simulink model "datafusion_realdata"  (R2020b)
settings: Solver=VariableStepAuto  StartTime=0.0  StopTime=20.0  RelTol=1e-3
model workspace (MAT data in the model file):
  sample_time = 0.01
libraries: simulink x4
settings Model: Creator=tfpeng  LastModifiedBy=tfpeng

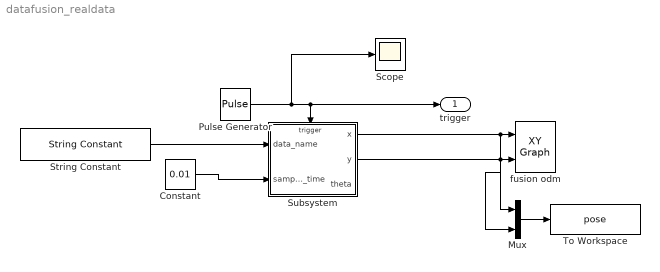
== system datafusion_realdata ==
  Constant : Constant  Value=0.01
  Mux : Mux  Inputs=2
  Pulse Generator : DiscretePulseGenerator  PulseType=Time based  Period=0.001  PulseWidth=50
  Scope : Scope
  String Constant : StringConstant  String="\"debug_output_2023-09-19_08:02:57.dat\""
  Subsystem : Subsystem
  To Workspace : ToWorkspace  VariableName=pose  SampleTime=-1
      settings: Save2DSignal=2-D array (concatenate along first dimension)
  fusion odm : simulink/Sinks/XY Graph  xmin=-5  xmax=5  ymin=-5  ymax=5  st=-1
  trigger : Outport
  wires:
  Pulse Generator/1 -> Scope/1, trigger/1, Subsystem/Trigger
  String Constant/1 -> Subsystem/1(data_name)
  Constant/1 -> Subsystem/2(sample_time)
  Subsystem/2(y) -> Mux/2, fusion odm/2
  Subsystem/1(x) -> Mux/1, fusion odm/1
  Mux/1 -> To Workspace/1

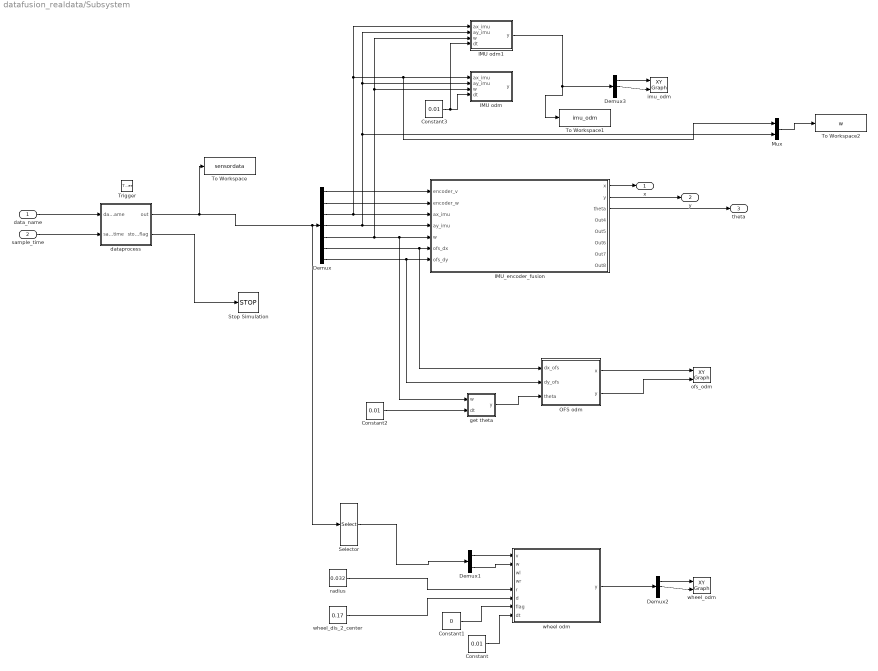
== system datafusion_realdata/Subsystem ==
  data_name : Inport
  sample_time : Inport  Port=2
  Trigger : TriggerPort  VariantControl=Variant  PortDimensions=1
  Constant : Constant  Value=0.01
  Constant1 : Constant  Value=0
  Constant2 : Constant  Value=0.01
  Constant3 : Constant  Value=0.01
  Demux : Demux  Outputs=7
  Demux1 : Demux  Outputs=2
  Demux2 : Demux  Outputs=3
  Demux3 : Demux  Outputs=3
  IMU odm : MATLAB Function  TreatAsAtomicUnit=on
  IMU odm1 : MATLAB Function  TreatAsAtomicUnit=on
  IMU_encoder_fusion : Subsystem
  Mux : Mux  Inputs=2
  OFS odm : Subsystem
  Selector : Selector  InputPortWidth=7  IndexOptions=Index vector (dialog)  Indices=[1 2]  OutputSizes=1
  Stop Simulation : Stop
  To Workspace : ToWorkspace  VariableName=sensordata  SampleTime=-1
      settings: Save2DSignal=2-D array (concatenate along first dimension)
  To Workspace1 : ToWorkspace  VariableName=imu_odm  SampleTime=-1
      settings: Save2DSignal=2-D array (concatenate along first dimension)
  To Workspace2 : ToWorkspace  VariableName=w  SampleTime=-1
      settings: Save2DSignal=2-D array (concatenate along first dimension)
  dataprocess : MATLAB Function  TreatAsAtomicUnit=on
  get theta : MATLAB Function  TreatAsAtomicUnit=on
  imu_odm : simulink/Sinks/XY Graph  xmin=-10  xmax=10  ymin=-10  ymax=10  st=-1
  ofs_odm : simulink/Sinks/XY Graph  xmin=-5  xmax=5  ymin=-5  ymax=5  st=-1
  radius : Constant  Value=0.032
  wheel odm : MATLAB Function  TreatAsAtomicUnit=on
  wheel_dis_2_center : Constant  Value=0.17
  wheel_odm : simulink/Sinks/XY Graph  xmin=-5  xmax=5  ymin=-5  ymax=5  st=-1
  x : Outport
  y : Outport  Port=2
  theta : Outport  Port=3
  wires:
  data_name/1 -> dataprocess/1(data_name)
  sample_time/1 -> dataprocess/2(sample_time)
  Demux/2 -> IMU_encoder_fusion/2(encoder_w)
  Demux/4 -> IMU odm1/2(ay_imu), IMU odm/2(ay_imu), Mux/2, IMU_encoder_fusion/4(ay_imu)
  Demux/3 -> IMU odm1/1(ax_imu), Mux/1, IMU odm/1(ax_imu), IMU_encoder_fusion/3(ax_imu)
  Demux/7 -> OFS odm/2(dy_ofs), IMU_encoder_fusion/7(ofs_dy)
  dataprocess/1(out) -> To Workspace/1, Selector/1, Demux/1
  Demux/6 -> OFS odm/1(dx_ofs), IMU_encoder_fusion/6(ofs_dx)
  Demux/1 -> IMU_encoder_fusion/1(encoder_v)
  IMU_encoder_fusion/1(x) -> x/1
  IMU_encoder_fusion/2(y) -> y/1
  IMU_encoder_fusion/3(theta) -> theta/1
  dataprocess/2(stop_flag) -> Stop Simulation/1
  wheel_dis_2_center/1 -> wheel odm/6(d)
  radius/1 -> wheel odm/5(r)
  Selector/1 -> Demux1/1
  Demux1/1 -> wheel odm/1(v)
  Demux1/2 -> wheel odm/2(w)
  Constant/1 -> wheel odm/8(dt)
  wheel odm/1(y) -> Demux2/1
  Demux2/1 -> wheel_odm/1
  Demux2/2 -> wheel_odm/2
  Constant1/1 -> wheel odm/7(flag)
  Constant2/1 -> get theta/2(dt)
  OFS odm/1(x) -> ofs_odm/1
  OFS odm/2(y) -> ofs_odm/2
  Demux/5 -> IMU odm1/3(w), IMU odm/3(w), get theta/1(w), IMU_encoder_fusion/5(w)
  get theta/1(y) -> OFS odm/3(theta)
  Constant3/1 -> IMU odm1/4(dt), IMU odm/4(dt)
  Demux3/2 -> imu_odm/2
  Demux3/1 -> imu_odm/1
  Mux/1 -> To Workspace2/1
  IMU odm1/1(y) -> To Workspace1/1, Demux3/1

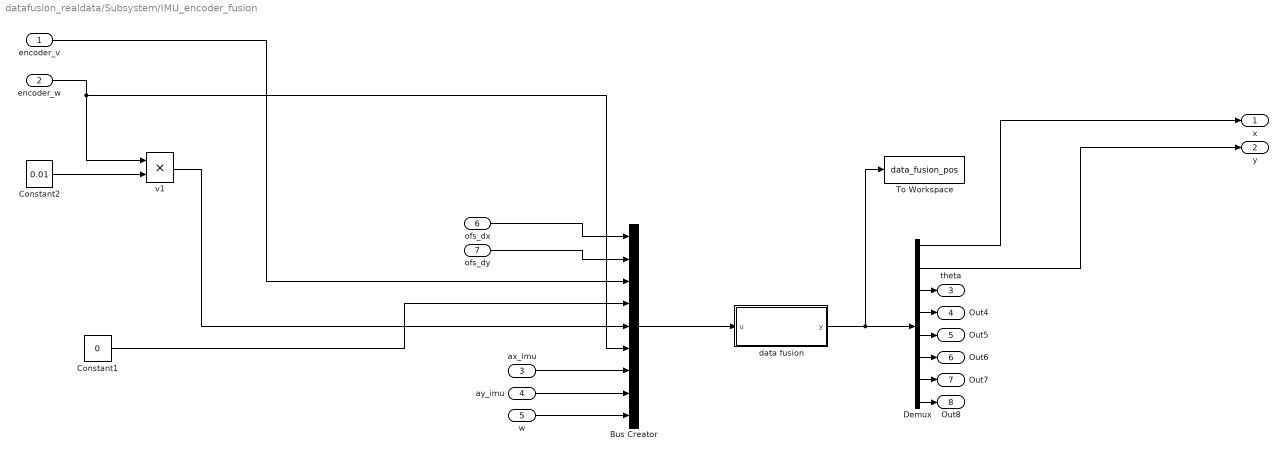
== system datafusion_realdata/Subsystem/IMU_encoder_fusion ==
  encoder_v : Inport
  encoder_w : Inport  Port=2
  ax_imu : Inport  Port=3
  ay_imu : Inport  Port=4
  w : Inport  Port=5
  ofs_dx : Inport  Port=6
  ofs_dy : Inport  Port=7
  Bus Creator : BusCreator  Inputs=9
  Constant1 : Constant  Value=0
  Constant2 : Constant  Value=0.01
  Demux : Demux  Outputs=8
  To Workspace : ToWorkspace  VariableName=data_fusion_pos  SampleTime=-1
      settings: Save2DSignal=2-D array (concatenate along first dimension)
  data fusion : Subsystem  TreatAsAtomicUnit=on
  v1 : Product
  x : Outport
  y : Outport  Port=2
  theta : Outport  Port=3
  Out4 : Outport  Port=4
  Out5 : Outport  Port=5
  Out6 : Outport  Port=6
  Out7 : Outport  Port=7
  Out8 : Outport  Port=8
  wires:
  Demux/7 -> Out7/1
  Demux/8 -> Out8/1
  Demux/2 -> y/1
  ax_imu/1 -> Bus Creator/7
  Demux/3 -> theta/1
  w/1 -> Bus Creator/9
  encoder_v/1 -> Bus Creator/3
  ay_imu/1 -> Bus Creator/8
  data fusion/1(y) -> To Workspace/1, Demux/1
  Demux/4 -> Out4/1
  Demux/1 -> x/1
  Demux/5 -> Out5/1
  Bus Creator/1 -> data fusion/1(u)
  Demux/6 -> Out6/1
  ofs_dx/1 -> Bus Creator/1
  ofs_dy/1 -> Bus Creator/2
  Constant2/1 -> v1/2
  encoder_w/1 -> Bus Creator/6, v1/1
  v1/1 -> Bus Creator/5
  Constant1/1 -> Bus Creator/4

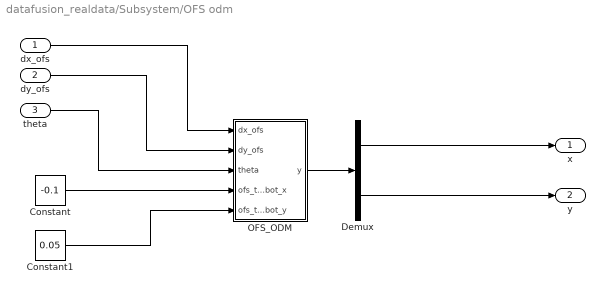
== system datafusion_realdata/Subsystem/OFS odm ==
  dx_ofs : Inport
  dy_ofs : Inport  Port=2
  theta : Inport  Port=3
  Constant : Constant  Value=-0.1
  Constant1 : Constant  Value=0.05
  Demux : Demux  Outputs=2
  OFS_ODM : MATLAB Function  TreatAsAtomicUnit=on
  x : Outport
  y : Outport  Port=2
  wires:
  Demux/2 -> y/1
  Demux/1 -> x/1
  theta/1 -> OFS_ODM/3(theta)
  dx_ofs/1 -> OFS_ODM/1(dx_ofs)
  OFS_ODM/1(y) -> Demux/1
  dy_ofs/1 -> OFS_ODM/2(dy_ofs)
  Constant/1 -> OFS_ODM/4(ofs_to_robot_x)
  Constant1/1 -> OFS_ODM/5(ofs_to_robot_y)

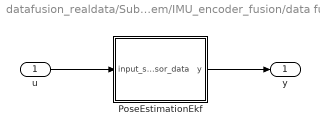
== system datafusion_realdata/Subsystem/IMU_encoder_fusion/data fusion ==
  u : Inport
  PoseEstimationEkf : MATLAB Function  TreatAsAtomicUnit=on
  y : Outport
  wires:
  u/1 -> PoseEstimationEkf/1(input_sensor_data)
  PoseEstimationEkf/1(y) -> y/1

== matlab function datafusion_realdata/Subsystem/wheel odm ==
  data: v input; y output; w input; wl input; wr input; r input; d input; flag input; dt input
function y = wheelodm( v,w,wl,wr,r,d,flag,dt)
persistent pos last_pos;
if isempty(pos)
   pos=zeros(3,1);%x,y,theta 
   last_pos=pos;
end
if flag==0
   %use v,w 
   vx=v*cos(pos(3));
   vy=v*sin(pos(3));
   dx=vx*dt;
   dy=vy*dt;
   dtheta=w*dt;
   pos=pos+[dx;dy;dtheta];
    
else
    %use wl,wr
    pos=zeros(3,1);%x,y,theta
    
end
y = pos;

== matlab function datafusion_realdata/Subsystem/dataprocess ==
  data: data_name input; out output; sample_time input; stop_flag output
function [out,stop_flag]= realdata_read(data_name,sample_time)
coder.extrinsic('realdata_read_callback');
out=[0,0,0,0,0,0,0];
stop_flag=0;
out=realdata_read_callback(data_name,sample_time);
if sum(out)==-7
    stop_flag=1;
end
% persistent fid;
% filepath="/home/tfpeng/work/other/TFwork/code/mat/car_simulation/";
% if isempty(fid)
%     fid=fopen(filepath+data_name,'r');
% end
% starttim=0;
% wheel_data=[];
% imu_data=[];
% ofs_data=[];
% 
% while 1
%     line=fgetl(fid);
%     newarr=split(line,': ');
%     rawdataarr=split(newarr(2)," ");
%     sensor_type=newarr{1};
%     rawdata=str2double(rawdataarr);
%     tim=rawdata(1);
%     if starttim==0
%         starttim=tim;
%     elseif contains(sensor_type,"wheel")
%        wheel_data=[wheel_data;[rawdata(1),rawdata(2)]];
%     elseif contains(sensor_type,"imu")
%        imu_data=[imu_data;[rawdata(1),rawdata(2),rawdata(3),rawdata(4),rawdata(5),rawdata(6)]]
%     elseif contains(sensor_type,"ofs")
%        ofs_data=[ofs_data;[rawdata(1),rawdata(2),rawdata(3),rawdata(4),rawdata(5)]]
%     end
%     
%     
%     if tim-starttim>=sample_time
%        break; 
%     end
%     
% end
% wheel_data_out=mean(wheel_data,1);
% imu_data_out=mean(imu_data,1);
% ofs_data_out=mean(ofs_data,1);

% out=[wheel_data_out,imu_data_out,ofs_data_out(1),ofs_data_out(2)];

== matlab function datafusion_realdata/Subsystem/IMU_encoder_fusion/data fusion/PoseEstimationEkf ==
  data: input_sensor_data input; y output
function y = PoseEstimationEkf(input_sensor_data)
persistent state_variable_current state_variable_last P Q counter vx_imu vy_imu vx_imu_last vy_imu_last;
if isempty(state_variable_current)
        state_variable_current=zeros(8,1);%[xt,yt,theta_t,vxt,vyt,wt,axt,ayt]
        state_variable_last=zeros(8,1);
        Q=diag([0.1, 0.1, 0.1,0.1, 0.1, 0.1, 0.1, 0.1]);
        P=Q;
        counter=0;
        vx_imu=0; 
        vy_imu=0;
        vx_imu_last=0;
        vy_imu_last=0;
end

%%    predict
dt=0.01;
A=[[1, 0, 0, dt, 0, 0, 0, 0]
  [0, 1, 0, 0, dt, 0, 0, 0]
  [0, 0, 1, 0, 0, dt, 0, 0]
  [0, 0, 0, 1, 0, 0, 0, 0]
  [0, 0, 0, 0, 1, 0, 0, 0]
  [0, 0, 0, 0, 0, 1, 0, 0]
  [0, 0, 0, 0, 0, 0, 0, 0]
  [0, 0, 0, 0, 0, 0, 0, 0]];
state_variable_current=A*state_variable_current;
P=A*P*A'+Q;

%%    update
theta=state_variable_current(3);
theta_last=state_variable_last(3);
vx=state_variable_current(4);
vy=state_variable_current(5);
ax=state_variable_current(7);
ay=state_variable_current(8);
dx=state_variable_current(1)-state_variable_last(1);
dy=state_variable_current(2)-state_variable_last(2);
w=state_variable_current(6);
dtheta=theta-theta_last;
v=vx*cos(theta)+vy*sin(theta);
vr=vx*sin(theta)-vy*cos(theta);
dd=sqrt(dx^2+dy^2);
% ax_imu=ax*cos(theta)+ay*sin(theta);
% ay_imu=-ax*sin(theta)+ay*cos(theta);

dx_ofs=dd*cos(dtheta/2);
dy_ofs=dd*sin(dtheta/2);

% ofs 
ofs_pos_robot=[-0.115;0.085];
rotation_matrix_last_robot_pose=[[cos(theta_last),-sin(theta_last)];
    [sin(theta_last),cos(theta_last)]];

rotation_matrix_current_robot_pose=[[cos(theta),-sin(theta)];
    [sin(theta),cos(theta)]];
last_robot_xy=[state_variable_last(1);state_variable_last(2)];
current_robot_xy=[state_variable_current(1);state_variable_current(2)];
temp2=ofs_pos_robot(1)*sin(theta)+ofs_pos_robot(2)*cos(theta);
temp3=ofs_pos_robot(1)*cos(theta)-ofs_pos_robot(2)*sin(theta);

%% all sensor data fusion ofs input distance
% H=[[cos(theta_last),sin(theta_last),cos(theta_last)*(-temp2)+temp3*sin(theta_last),0,0,0,0,0]
%    [-sin(theta_last),cos(theta_last),temp2*sin(theta_last)+temp3*cos(theta_last),0,0,0,0,0]
%    [0, 0, -vx*sin(theta)+vy*cos(theta), cos(theta), sin(theta), 0, 0, 0]
%    [0, 0, vx*cos(theta)+vy*sin(theta), sin(theta), -cos(theta), 0, 0, 0]
%    [0, 0, 1, 0, 0, 0, 0, 0]
%    [0, 0, 0, 0, 0, 1, 0, 0]
%    [0, 0, -ax*sin(theta)+ay*cos(theta), 0, 0, 0, cos(theta), sin(theta)]
%    [0, 0, -ax*cos(theta)-ay*sin(theta), 0, 0, 0, -sin(theta), cos(theta)]
%    [0, 0, 0, 0, 0, 1, 0, 0]
%    [0, 0, 1, 0, 0, 0, 0, 0]];
% Z_ofs=rotation_matrix_last_robot_pose\(current_robot_xy-last_robot_xy+rotation_matrix_current_robot_pose*ofs_pos_robot)-ofs_pos_robot;
% Z=[Z_ofs;v;vr;dtheta; w;ax_imu; ay_imu;w;dtheta];
% R = diag([0.001,0.001,0.00001,0.00001,0.00001,0.00001,0.0002,0.0002,0.0002,0.0002]);
% encoder_input_sensor_data=input_sensor_data(3:6);
% imu_input_sensor_data=[input_sensor_data(7:9);input_sensor_data(9)*dt];
% ofs_input_sensor_data=input_sensor_data(1:2);
% 
% temp_input_data=[ofs_input_sensor_data;encoder_input_sensor_data;imu_input_sensor_data];
% error=temp_input_data-Z;

%%
%% all sensor data fusion ofs input velocity
% dt=0.01;
% phi=atan(ofs_pos_robot(1)/ofs_pos_robot(2));
% l=(ofs_pos_robot'*ofs_pos_robot)^0.5;
% extern_veloctiy=[w*l*sin(phi+pi/2);w*l*sin(phi)*cos(phi+pi/2)];
% H=[[0,0,-vx*sin(theta)+vy*cos(theta)-w*l*cos(phi+pi/2-theta),cos(theta),sin(theta),l*sin(phi+pi/2-theta),0,0]
%     [0,0,-vx*cos(theta)-vy*sin(theta)+w*l*sin(phi+pi/2-theta),-sin(theta),cos(theta),l*cos(phi+pi/2-theta),0,0]
%    [0, 0, -vx*sin(theta)+vy*cos(theta), cos(theta), sin(theta), 0, 0, 0]
%    [0, 0, vx*cos(theta)+vy*sin(theta), sin(theta), -cos(theta), 0, 0, 0]
%    [0, 0, 1, 0, 0, 0, 0, 0]
%    [0, 0, 0, 0, 0, 1, 0, 0]
%    [0, 0, -ax*sin(theta)+ay*cos(theta), 0, 0, 0, cos(theta), sin(theta)]
%    [0, 0, -ax*cos(theta)-ay*sin(theta), 0, 0, 0, -sin(theta), cos(theta)]
%    [0, 0, 0, 0, 0, 1, 0, 0]
%    [0, 0, 1, 0, 0, 0, 0, 0]];
% Z_ofs=rotation_matrix_current_robot_pose\[vx;vy]+rotation_matrix_current_robot_pose*extern_veloctiy;
% Z=[Z_ofs;v;vr;dtheta; w;ax_imu; ay_imu;w;dtheta];
% R = diag([0.001,0.001,0.001,0.001,0.001,0.001,0.0002,0.0002,0.0002,0.0002]);
% encoder_input_sensor_data=input_sensor_data(3:6);
% imu_input_sensor_data=[input_sensor_data(7:9);input_sensor_data(9)*dt];
% ofs_input_sensor_data=input_sensor_data(1:2);
% 
% temp_input_data=[ofs_input_sensor_data;encoder_input_sensor_data;imu_input_sensor_data];
% error=temp_input_data-Z;
%% just wheel encoder fusion  --debug ok
% H=[[0, 0, -vx*sin(theta)+vy*cos(theta), cos(theta), sin(theta), 0, 0, 0]
%   [0, 0, vx*cos(theta)+vy*sin(theta), sin(theta), -cos(theta), 0, 0, 0]
%   [0, 0, 1, 0, 0, 0, 0, 0]
%   [0, 0, 0, 0, 0, 1, 0, 0]];
% Z=[v,vr,dtheta, w]';
% R = diag([0.001, 0.001,0.001,0.001]);
% temp_input_sensor_data=input_sensor_data(3:6);
% error=temp_input_sensor_data-Z;

%% just IMU fusion    --debug ok
% H=[[0, 0, -ax*sin(theta)+ay*cos(theta), 0, 0, 0, cos(theta), sin(theta)]
%   [0, 0, -ax*cos(theta)-ay*sin(theta), 0, 0, 0, -sin(theta), cos(theta)]
%   [0, 0, 0, 0, 0, 1, 0, 0]
%   [0, 0, 1, 0, 0, 0, 0, 0]];
% Z=[ax_imu, ay_imu,w,dtheta]';
% R = diag([0.001,0.001,0.001,0.001]);
% %[ax_imu,ay_imu,w]
% input_sensor_data=[input_sensor_data(7:9);input_sensor_data(9)*dt];
% error=input_sensor_data-Z;

%% just IMU fusion new version 
% v_imu=rotation_matrix_current_robot_pose\[vx;vy];
% temp=v_imu-[vx_imu_last;vy_imu_last];
% a_imu=temp/dt;
% ax_imu=a_imu(1,1);
% ay_imu=a_imu(2,1);
% vx_imu_last=v_imu(1,1);
% vy_imu_last=v_imu(2,1);
% H=[[0, 0, (-vx*sin(theta)+vy*cos(theta))/dt, cos(theta)/dt, sin(theta)/dt, 0, 0, 0]
%   [0, 0, -(-vx*cos(theta)-vy*sin(theta))/dt, sin(theta)/dt, -cos(theta)/dt, 0, 0, 0]
%   [0, 0, 0, 0, 0, 1, 0, 0]
%   [0, 0, 1, 0, 0, 0, 0, 0]];
% Z=[ax_imu, -ay_imu,w,dtheta]';
% R = diag([0.001,0.001,0.001,0.001]);
% %[ax_imu,ay_imu,w]
% input_sensor_data=[input_sensor_data(7:9);input_sensor_data(9)*dt];
% error=input_sensor_data-Z;

%%  IMU wheel encoder 
v_imu=rotation_matrix_current_robot_pose\[vx;vy];
temp=v_imu-[vx_imu_last;vy_imu_last];
a_imu=temp/dt;
ax_imu=a_imu(1,1);
ay_imu=a_imu(2,1);
vx_imu_last=v_imu(1,1);
vy_imu_last=v_imu(2,1);
H=[[0, 0, -vx*sin(theta)+vy*cos(theta), cos(theta), sin(theta), 0, 0, 0]
  [0, 0, vx*cos(theta)+vy*sin(theta), sin(theta), -cos(theta), 0, 0, 0]
  [0, 0, 1, 0, 0, 0, 0, 0]
  [0, 0, 0, 0, 0, 1, 0, 0]
  [0, 0, (-vx*sin(theta)+vy*cos(theta))/dt, cos(theta)/dt, sin(theta)/dt, 0, 0, 0]
  [0, 0, -(-vx*cos(theta)-vy*sin(theta))/dt, sin(theta)/dt, -cos(theta)/dt, 0, 0, 0]
  [0, 0, 0, 0, 0, 1, 0, 0]
  [0, 0, 1, 0, 0, 0, 0, 0]];
Z=[v,vr,dtheta, w,ax_imu, -ay_imu,w,dtheta]';
R = diag([0.0001,0.0001,0.0001,0.0001,0.02,0.02,0.02,0.02]);
encoder_input_sensor_data=input_sensor_data(3:6);
imu_input_sensor_data=[input_sensor_data(7:9);input_sensor_data(9)*dt];
temp_input_data=[encoder_input_sensor_data;imu_input_sensor_data];
error=temp_input_data-Z;

%% correct update
temp_p=H*P*H'+R;
kalman_gain=(P*H')/(temp_p);
correct_value=kalman_gain*error;
state_variable_current=state_variable_current+correct_value;
P=P-kalman_gain*H*P;
state_variable_last=state_variable_current;
counter=counter+1;
y = state_variable_current;

== matlab function datafusion_realdata/Subsystem/get theta ==
  data: w input; y output; dt input
function y = fcn(w,dt)
persistent theta last_w;
if isempty(last_w)
    theta=0;
    last_w=0;
end
dtheta=(w+last_w)*0.5*dt;
theta=theta+dtheta;
last_w=w;
y = theta;

== matlab function datafusion_realdata/Subsystem/IMU odm ==
  data: ax_imu input; y output; ay_imu input; w input; dt input
function y = fcn(ax_imu,ay_imu,w,dt)
persistent pos vx_last vy_last ax_last ay_last w_last;
if isempty(pos)
    pos=zeros(3,1);
    vx_last=0;
    vy_last=0;
    ax_last=0;
    ay_last=0;
    w_last=0;
end

dtheta=(w+w_last)*0.5*dt;
ax=ax_imu*cos(pos(3)+dtheta)-ay_imu*sin(pos(3)+dtheta);
ddx=vx_last*dt+(ax+ax_last)*dt^2/4;

ay=ax_imu*sin(pos(3)+dtheta)+ay_imu*cos(pos(3)+dtheta);
ddy=vy_last*dt+(ay+ay_last)*dt^2/4;

% ax=ax_imu*cos(pos(3)+dtheta)+ay_imu*sin(pos(3)+dtheta);
% ddx=vx_last*dt+(ax+ax_last)*dt^2/4;
% 
% ay=ax_imu*sin(pos(3)+dtheta)-ay_imu*cos(pos(3)+dtheta);
% ddy=vy_last*dt+(ay+ay_last)*dt^2/4;

vx_last=vx_last+(ax+ax_last)*dt/2;
vy_last=vy_last+(ay+ay_last)*dt/2;
ax_last=ax;
ay_last=ay;
w_last=w;
pos=pos+[ddx;ddy;dtheta];
y = pos;

== matlab function datafusion_realdata/Subsystem/OFS odm/OFS_ODM ==
  data: dx_ofs input; y output; dy_ofs input; theta input; ofs_to_robot_x input; ofs_to_robot_y input
function y = OfsOdm(dx_ofs,dy_ofs,theta,ofs_to_robot_x,ofs_to_robot_y)
persistent  current_robot_xy last_robot_xy  last_robot_theta;
if isempty(last_robot_xy)
   last_robot_xy=[0;0];
   last_robot_theta=0;
end

current_robot_theta=theta;
current_ofs_pose=[ofs_to_robot_x;ofs_to_robot_y];


rotation_matrix_last_robot_pose=[[cos(last_robot_theta),-sin(last_robot_theta)];
    [sin(last_robot_theta),cos(last_robot_theta)]];

rotation_matrix_current_robot_pose=[[cos(current_robot_theta),-sin(current_robot_theta)];
    [sin(current_robot_theta),cos(current_robot_theta)]];
dfos=[dx_ofs;dy_ofs];
current_robot_xy=rotation_matrix_last_robot_pose*(dfos+current_ofs_pose)+last_robot_xy-rotation_matrix_current_robot_pose*current_ofs_pose;
last_robot_xy=current_robot_xy;
last_robot_theta=current_robot_theta;
y = [current_robot_xy];

== matlab function datafusion_realdata/Subsystem/IMU odm1 ==
  data: ax_imu input; y output; ay_imu input; w input; dt input
function y = fcn(ax_imu,ay_imu,w,dt)
persistent pos vx_last vy_last  w_last vx_imu vy_imu vx_imu_last vy_imu_last;
if isempty(pos)
    pos=zeros(3,1);
    vx_last=0;
    vy_last=0;

    w_last=0;
    vx_imu=0;
    vy_imu=0;
    vx_imu_last=0;
    vy_imu_last=0;
end

dtheta=(w+w_last)*0.5*dt;
theta=pos(3)+dtheta;

vx_imu=vx_imu+ax_imu*dt;
vy_imu=vy_imu+ay_imu*dt;


ddx_imu=(vx_imu+vx_imu_last)*dt/2;
ddy_imu=(vy_imu+vy_imu_last)*dt/2;
% 
% ddx=ddx_imu*cos(theta)-ddx_imu*sin(theta);
% ddy=ddy_imu*sin(theta)+ddy_imu*cos(theta);


vx=vx_imu*cos(theta)-vy_imu*sin(theta);
vy=vx_imu*sin(theta)+vy_imu*cos(theta);
ddx=(vx+vx_last)*dt/2;
ddy=(vy+vy_last)*dt/2;
vx_last=vx;
vy_last=vy;


w_last=w;
vx_imu_last=vx_imu;
vy_imu_last=vy_imu;
pos=pos+[ddx;ddy;dtheta];
y = pos;
